simulink model "pendulum"  (R2018a)
settings: Solver=VariableStepAuto  StartTime=0.0  StopTime=100  MaxStep=0.01  RelTol=1e-3
values from neighbouring files (symbols this model uses):
  b = [0.1, 0.5, 1]    [init.m]
  g = 9.8    [init.m]
  J = m*l^2    (= 1)    [init.m]
  l = 1    [init.m]
  m = 1    [init.m]
libraries: simulink_extras x1
settings Model: Creator=Asus  LastModifiedBy=Asus

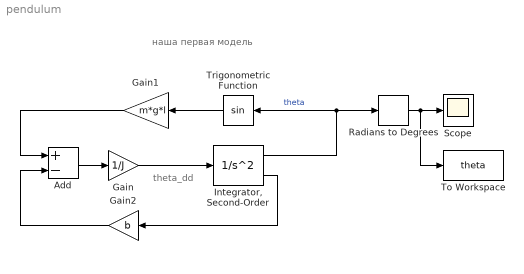
== system pendulum ==
  note: theta_dd
  note: наша первая модель
  Add : Sum  Inputs=+-
  Gain : Gain  Gain=1/J
  Gain1 : Gain  Gain=m*g*l
  Gain2 : Gain  Gain=b
  "Integrator, Second-Order" : SecondOrderIntegrator  ICX=0.01
  Radians to Degrees : simulink_extras/Transformations/Radians to Degrees
  Scope : Scope
  To Workspace : ToWorkspace  VariableName=theta  SampleTime=-1
  Trigonometric Function : Trigonometry
  wires:
  Gain/1 -> "Integrator, Second-Order"/1
  "Integrator, Second-Order"/1 -> Trigonometric Function/1, Radians to Degrees/1  "theta"
  Trigonometric Function/1 -> Gain1/1
  Add/1 -> Gain/1
  Gain1/1 -> Add/1
  Gain2/1 -> Add/2
  "Integrator, Second-Order"/2 -> Gain2/1
  Radians to Degrees/1 -> To Workspace/1, Scope/1
